simulink model "PubIfDecisionLM_MDL"  (R2020b)
settings: configuration reference "DspaceConfig" (kept outside this file)
PostLoadFcn:
  | if any(exist('dsrtsu_mdlpostloadfcn', 'file') ~= 0), dsrtsu_mdlpostloadfcn('Execute', bdroot); end
InitFcn:
  | , if any(exist('dsmpb_private', 'file') ~= 0), dsmpb_private('dsmpb_mdlclblib', 'Init', bdroot); end,
undefined symbols (not defined in the file or in its folder): OFM_OBJ_FUSIONTYPE_E, OFM_OBJ_MOVINGSTATE_E, OFM_OBJ_ORIENTATION_E, OFM_OBJ_TYPE_E, P_LM_Cyc, P_LM_EMLHistKapRcdBufSize, P_LM_EMLHistTrajBaseDis, P_LM_EMLHistTrajPNum, P_LM_EMLKapCorrMaxThre, P_LM_EMLMinKapThre, P_LM_EMLPathDisDiffThre, P_LM_EMLQuaFiltPar, P_LM_EMLTurnActKapThre, P_LM_EMLValidQuaThre, P_LM_FntPath1Disgap, P_LM_FntPath1MinDis, P_LM_FntPath1Timegap, P_LM_FntPath2Disgap, P_LM_FntPath2MinDis, P_LM_FntPath2Timegap, P_LM_FntPath3Disgap, P_LM_FntPath3MinDis, P_LM_FntPath3Timegap, P_LM_FusBLParFiltP, P_LM_FusEVDifC2Thre, P_LM_FusEVOPath1AllVSLDisThre, P_LM_FusEVOPath1AllVSLLostNumThre, P_LM_FusEVOPath1AllVSLQuaThre, P_LM_FusEVOPath1OTLFacNLC, P_LM_FusOTLQuaThre, P_LM_FusOTLSW, P_LM_FusParC0Index, P_LM_FusParC1Index, P_LM_FusParC2Index, P_LM_FusParC3Index, P_LM_FusVSLQuaThre, P_LM_FusVSLSW, P_LM_FusVSLValidSteerWheerAngThre, P_LM_FusVSLValidVxvThre, P_LM_LaneWidth, P_LM_OTLBufTPInfoEvaFactor, P_LM_OTLObjNum, P_LM_OTLObjSelectAgeThre, P_LM_OTLObjSelectDxAssessVx, P_LM_OTLObjSelectDxThre, P_LM_OTLObjSelectVxThre, P_LM_OTLObjSelectVyAssessDx, P_LM_OTLObjSelectVyThre, P_LM_OTLTrajPntBaseDis, P_LM_OTLTrajStdThre, P_LM_VSLAvailLineNum, P_LM_VSLBLSDiffThre, P_LM_VSLBLSDisRatio, P_LM_VSLFusBLParFiltP_C1, P_LM_VSLFusBLParFiltP_C2, P_LM_VSLFusBLParFiltP_C3, P_LM_VSLFusBLParFiltP_Quality, P_LM_VSLHistTrajBaseDis, P_LM_VSLHistTrajPNum, P_LM_VSLLCC0diff ... (+18)
libraries: simulink x145, LM_LIB x43
(part 8 of 24)

== system PubIfDecisionLM_MDL/Subsystem2/LM_Fusion1/LM_FusRatioCalc/LM_Fusion_EMLOnly/LM_FusEMLAndVSLRatioCalc ==
  Bus Creator : BusCreator  Inputs=15  OutDataTypeStr=Bus: LM_FusFntPathKInfoBus  NonVirtualBus=on
  Bus Creator1 : BusCreator  Inputs=6  OutDataTypeStr=Bus: LM_FusRearPathKInfoBus  NonVirtualBus=on
  Constant : Constant  OutDataTypeStr=single
  Constant1 : Constant  OutDataTypeStr=single
  Constant{3..14} (12 alike) : Constant  Value=0  OutDataTypeStr=single
  Constant2 : Constant  OutDataTypeStr=single
  LM_Fusion_RearPathK : Subsystem
  LM_FusFntPathK : Outport
  LM_FusRearPathK : Outport  Port=2
  wires:
  Constant9/1 -> Bus Creator/9  "LM_FusFntPath2RELK"
  Constant1/1 -> Bus Creator/6  "LM_FusFntPath2EMLK"
  Constant6/1 -> Bus Creator/5  "LM_FusFntPath1MALK"
  Constant10/1 -> Bus Creator/10  "LM_FusFntPath2MALK"
  Constant7/1 -> Bus Creator/7  "LM_FusFntPath2VSLK"
  Constant8/1 -> Bus Creator/8  "LM_FusFntPath2OTLK"
  Constant/1 -> Bus Creator/1  "LM_FusFntPath1EMLK"
  Constant3/1 -> Bus Creator/2  "LM_FusFntPath1VSLK"
  Constant14/1 -> Bus Creator/14  "LM_FusFntPath3RELK"
  Constant12/1 -> Bus Creator/12  "LM_FusFntPath3VSLK"
  Constant4/1 -> Bus Creator/3  "LM_FusFntPath1OTLK"
  Constant11/1 -> Bus Creator/15  "LM_FusFntPath3MALK"
  Constant5/1 -> Bus Creator/4  "LM_FusFntPath1RELK"
  Constant13/1 -> Bus Creator/13  "LM_FusFntPath3OTLK"
  Constant2/1 -> Bus Creator/11  "LM_FusFntPath3EMLK"
  Bus Creator1/1 -> LM_FusRearPathK/1  "LM_FusRearPathK"
  LM_Fusion_RearPathK/1(LM_FusRearPath1VSLK) -> Bus Creator1/1
  LM_Fusion_RearPathK/4(LM_FusRearPath1EMLK) -> Bus Creator1/4
  LM_Fusion_RearPathK/3(LM_FusRearPath3VSLK) -> Bus Creator1/3
  LM_Fusion_RearPathK/2(LM_FusRearPath2VSLK) -> Bus Creator1/2
  LM_Fusion_RearPathK/5(LM_FusRearPath2EMLK) -> Bus Creator1/5
  LM_Fusion_RearPathK/6(LM_FusRearPath3EMLK) -> Bus Creator1/6
  Bus Creator/1 -> LM_FusFntPathK/1  "LM_FusFntPathK"

== system PubIfDecisionLM_MDL/Subsystem2/LM_Fusion1/LM_FusRatioCalc/LM_Fusion_EO/LM_FusBaseLineC0Info ==
  LM_VSLLLC0Adju : Inport
  LM_VSLLRC0Adju : Inport  Port=2
  LM_VSLRLC0Adju : Inport  Port=3
  LM_VSLRRC0Adju : Inport  Port=4
  Signal Conversion{,1..3} (4 alike) : SignalConversion  OverrideOpt=off
  LM_LLC0 : Outport
  LM_LRC0 : Outport  Port=2
  LM_RLC0 : Outport  Port=3
  LM_RRC0 : Outport  Port=4
  wires:
  Signal Conversion3/1 -> LM_RRC0/1  "LM_RRC0"
  Signal Conversion2/1 -> LM_RLC0/1  "LM_RLC0"
  Signal Conversion1/1 -> LM_LRC0/1  "LM_LRC0"
  Signal Conversion/1 -> LM_LLC0/1  "LM_LLC0"
  LM_VSLRRC0Adju/1 -> Signal Conversion3/1
  LM_VSLRLC0Adju/1 -> Signal Conversion2/1
  LM_VSLLRC0Adju/1 -> Signal Conversion1/1
  LM_VSLLLC0Adju/1 -> Signal Conversion/1

== system PubIfDecisionLM_MDL/Subsystem2/LM_Fusion1/LM_FusRatioCalc/LM_Fusion_EO/LM_FusEVORatioCalc ==
  DIR_BUS : Inport
  LM_EML : Inport  Port=2
  LM_OTL : Inport  Port=3
  LM_Com : Inport  Port=4
  LM_VIE_BUS : Inport  Port=5
  Bus Creator : BusCreator  Inputs=15  OutDataTypeStr=Bus: LM_FusFntPathKInfoBus  NonVirtualBus=on
  Bus Creator1 : BusCreator  Inputs=6  OutDataTypeStr=Bus: LM_FusRearPathKInfoBus  NonVirtualBus=on
  Bus Selector : BusSelector  OutputSignals=LM_EMLFntPath1Quality,LM_EMLFntPath2Quality,LM_EMLFntPath3Quality
  Bus Selector1 : BusSelector  OutputSignals=LM_DIRTurnLeftValid,LM_DIRTurnRightValid,DIR_LC2LeValid,DIR_LC2RigValid
  Bus Selector3 : BusSelector  OutputSignals=LM_OTLFntPath1Qulity,LM_OTLFntPath2Qulity,LM_OTLFntPath3Qulity
  Bus Selector4 : BusSelector  OutputSignals=vxvRefMs
  LM_Fusion_FntPathK : Subsystem
  LM_Fusion_RearPathK : Subsystem
  Signal Conversion{,1..14} (15 alike) : SignalConversion  OverrideOpt=off
  LM_FusFntPathK : Outport
  LM_FusRearPathK : Outport  Port=2
  wires:
  Bus Selector4/1 -> LM_Fusion_FntPathK/7(vxvRefMs)  "<vxvRefMs>"
  LM_VIE_BUS/1 -> Bus Selector4/1
  Bus Selector3/3 -> LM_Fusion_FntPathK/6(LM_OTLFntPath3Qulity)  "<LM_OTLFntPath3Qulity>"
  Bus Selector3/2 -> LM_Fusion_FntPathK/5(LM_OTLFntPath2Qulity)  "<LM_OTLFntPath2Qulity>"
  Bus Selector3/1 -> LM_Fusion_FntPathK/4(LM_OTLFntPath1Qulity)  "<LM_OTLFntPath1Qulity>"
  Bus Selector/3 -> LM_Fusion_FntPathK/3(LM_EMLFntPath3Quality)  "<LM_EMLFntPath3Quality>"
  Bus Selector/2 -> LM_Fusion_FntPathK/2(LM_EMLFntPath2Quality)  "<LM_EMLFntPath2Quality>"
  Bus Selector/1 -> LM_Fusion_FntPathK/1(LM_EMLFntPath1Quality)  "<LM_EMLFntPath1Quality>"
  LM_OTL/1 -> Bus Selector3/1
  LM_EML/1 -> Bus Selector/1
  Bus Creator1/1 -> LM_FusRearPathK/1  "LM_FusRearPathK"
  LM_Fusion_RearPathK/1(LM_FusRearPath1VSLK) -> Bus Creator1/1
  LM_Fusion_RearPathK/4(LM_FusRearPath1EMLK) -> Bus Creator1/4
  LM_Fusion_RearPathK/3(LM_FusRearPath3VSLK) -> Bus Creator1/3
  LM_Fusion_RearPathK/2(LM_FusRearPath2VSLK) -> Bus Creator1/2
  LM_Fusion_RearPathK/5(LM_FusRearPath2EMLK) -> Bus Creator1/5
  LM_Fusion_RearPathK/6(LM_FusRearPath3EMLK) -> Bus Creator1/6
  Bus Creator/1 -> LM_FusFntPathK/1  "LM_FusFntPathK"
  LM_Fusion_FntPathK/1(LM_FusEOFntPath1EMLK) -> Signal Conversion/1
  LM_Fusion_FntPathK/2(LM_FusEOFntPath1VSLK) -> Signal Conversion1/1
  LM_Fusion_FntPathK/3(LM_FusEOFntPath1OTLK) -> Signal Conversion2/1
  LM_Fusion_FntPathK/4(LM_FusEOFntPath1RELK) -> Signal Conversion3/1
  LM_Fusion_FntPathK/5(LM_FusEOFntPath1MALK) -> Signal Conversion4/1
  LM_Fusion_FntPathK/6(LM_FusEOFntPath2EMLK) -> Signal Conversion5/1
  LM_Fusion_FntPathK/7(LM_FusEOFntPath2VSLK) -> Signal Conversion6/1
  LM_Fusion_FntPathK/8(LM_FusEOFntPath2OTLK) -> Signal Conversion7/1
  LM_Fusion_FntPathK/9(LM_FusEOFntPath2RELK) -> Signal Conversion8/1
  LM_Fusion_FntPathK/10(LM_FusEOFntPath2MALK) -> Signal Conversion9/1
  LM_Fusion_FntPathK/11(LM_FusEOFntPath3EMLK) -> Signal Conversion10/1
  LM_Fusion_FntPathK/12(LM_FusEOFntPath3VSLK) -> Signal Conversion11/1
  LM_Fusion_FntPathK/13(LM_FusEOFntPath3OTLK) -> Signal Conversion12/1
  LM_Fusion_FntPathK/14(LM_FusEOFntPath3RELK) -> Signal Conversion13/1
  LM_Fusion_FntPathK/15(LM_FusEOFntPath3MALK) -> Signal Conversion14/1
  Signal Conversion/1 -> Bus Creator/1  "LM_FusFntPath1EMLK"
  Signal Conversion1/1 -> Bus Creator/2  "LM_FusFntPath1VSLK"
  Signal Conversion2/1 -> Bus Creator/3  "LM_FusFntPath1OTLK"
  Signal Conversion3/1 -> Bus Creator/4  "LM_FusFntPath1RELK"
  Signal Conversion4/1 -> Bus Creator/5  "LM_FusFntPath1MALK"
  Signal Conversion7/1 -> Bus Creator/8  "LM_FusFntPath2OTLK"
  Signal Conversion6/1 -> Bus Creator/7  "LM_FusFntPath2VSLK"
  Signal Conversion8/1 -> Bus Creator/9  "LM_FusFntPath2RELK"
  Signal Conversion9/1 -> Bus Creator/10  "LM_FusFntPath2MALK"
  Signal Conversion5/1 -> Bus Creator/6  "LM_FusFntPath2EMLK"
  Signal Conversion11/1 -> Bus Creator/12  "LM_FusFntPath3VSLK"
  Signal Conversion10/1 -> Bus Creator/11  "LM_FusFntPath3EMLK"
  Signal Conversion12/1 -> Bus Creator/13  "LM_FusFntPath3OTLK"
  Signal Conversion13/1 -> Bus Creator/14  "LM_FusFntPath3RELK"
  Signal Conversion14/1 -> Bus Creator/15  "LM_FusFntPath3MALK"
  DIR_BUS/1 -> Bus Selector1/1
  Bus Selector1/2 -> LM_Fusion_FntPathK/9(DIR_TurnRightValid)  "<LM_DIRTurnRightValid>"
  Bus Selector1/1 -> LM_Fusion_FntPathK/8(DIR_TurnLeftValid)  "<LM_DIRTurnLeftValid>"
  Bus Selector1/3 -> LM_Fusion_FntPathK/10(DIR_LC2LeValid)  "<DIR_LC2LeValid>"
  Bus Selector1/4 -> LM_Fusion_FntPathK/11(DIR_LC2RigValid)  "<DIR_LC2RigValid>"

== system PubIfDecisionLM_MDL/Subsystem2/LM_Fusion1/LM_FusRatioCalc/LM_Fusion_EV/LM_FusBaseLineC0Info ==
  LM_FusFntPathK : Inport
  LM_VSL : Inport  Port=2
  LM_EML : Inport  Port=3
  Bus Selector : BusSelector  OutputSignals=LM_VSLLLC0,LM_VSLLRC0,LM_VSLRLC0,LM_VSLRRC0
  Bus Selector1 : BusSelector  OutputSignals=LM_FusFntPath1EMLK
  Bus Selector2 : BusSelector  OutputSignals=LM_EMLLLC0,LM_EMLLRC0,LM_EMLRLC0,LM_EMLRRC0
  Constant : Constant  OutDataTypeStr=single
  If : If  IfExpression=u1 ~= 0
  If Action Subsystem : Subsystem  TreatAsAtomicUnit=on
  If Action Subsystem1 : Subsystem  TreatAsAtomicUnit=on
  Merge{,1..3} (4 alike) : Merge
  Relational Operator : RelationalOperator  Operator===  OutDataTypeStr=boolean  RndMeth=Simplest
  LM_LLC0 : Outport
  LM_LRC0 : Outport  Port=2
  LM_RLC0 : Outport  Port=3
  LM_RRC0 : Outport  Port=4
  wires:
  LM_FusFntPathK/1 -> Bus Selector1/1
  Bus Selector1/1 -> Relational Operator/1  "<LM_FusFntPath1EMLK>"
  Relational Operator/1 -> If/1
  If/1 -> If Action Subsystem/Action
  If/2 -> If Action Subsystem1/Action
  Bus Selector/1 -> If Action Subsystem1/1(LM_VSLLLC0Adju)  "<LM_VSLLLC0>"
  Bus Selector/2 -> If Action Subsystem1/2(LM_VSLLRC0Adju)  "<LM_VSLLRC0>"
  Bus Selector/3 -> If Action Subsystem1/3(LM_VSLRLC0Adju)  "<LM_VSLRLC0>"
  Bus Selector/4 -> If Action Subsystem1/4(LM_VSLRRC0Adju)  "<LM_VSLRRC0>"
  LM_VSL/1 -> Bus Selector/1
  Bus Selector2/1 -> If Action Subsystem/1(LM_EMLLLC0Adju)  "<LM_EMLLLC0>"
  Bus Selector2/2 -> If Action Subsystem/2(LM_EMLLRC0Adju)  "<LM_EMLLRC0>"
  Bus Selector2/3 -> If Action Subsystem/3(LM_EMLRLC0Adju)  "<LM_EMLRLC0>"
  Bus Selector2/4 -> If Action Subsystem/4(LM_EMLRRC0Adju)  "<LM_EMLRRC0>"
  LM_EML/1 -> Bus Selector2/1
  If Action Subsystem/1(LM_LLC0) -> Merge/1
  If Action Subsystem1/1(LM_LLC0) -> Merge/2
  If Action Subsystem/2(LM_LRC0) -> Merge1/1
  If Action Subsystem1/2(LM_LRC0) -> Merge1/2
  If Action Subsystem/3(LM_RLC0) -> Merge2/1
  If Action Subsystem1/3(LM_RLC0) -> Merge2/2
  If Action Subsystem/4(LM_RRC0) -> Merge3/1
  If Action Subsystem1/4(LM_RRC0) -> Merge3/2
  Merge/1 -> LM_LLC0/1  "LM_LLC0"
  Merge1/1 -> LM_LRC0/1  "LM_LRC0"
  Merge2/1 -> LM_RLC0/1  "LM_RLC0"
  Merge3/1 -> LM_RRC0/1  "LM_RRC0"
  Constant/1 -> Relational Operator/2

== system PubIfDecisionLM_MDL/Subsystem2/LM_Fusion1/LM_FusRatioCalc/LM_Fusion_EV/LM_FusEMLAndVSLRatioCalc ==
  LM_VIE_BUS : Inport
  LM_ComBus : Inport  Port=2
  DIR_BUS : Inport  Port=3
  LM_VSL : Inport  Port=4
  LM_EML : Inport  Port=5
  Bus Creator : BusCreator  Inputs=15  OutDataTypeStr=Bus: LM_FusFntPathKInfoBus  NonVirtualBus=on
  Bus Creator1 : BusCreator  Inputs=6  OutDataTypeStr=Bus: LM_FusRearPathKInfoBus  NonVirtualBus=on
  Bus Selector : BusSelector  OutputSignals=LM_VSLFntPath1Quality,LM_VSLFntPath2Quality,LM_VSLFntPath3Quality,LM_VSLFntPath1P,LM_VSLBaseDis
  Bus Selector1 : BusSelector  OutputSignals=LM_EMLFntPath1Quality,LM_EMLFntPath2Quality,LM_EMLFntPath3Quality,LM_EMLFntPath1P
  Bus Selector2 : BusSelector  OutputSignals=LM_ComLineLostNum
  Bus Selector3 : BusSelector  OutputSignals=LM_DIRTurnLeftValid,LM_DIRTurnRightValid,DIR_LC2LeValid,DIR_LC2RigValid
  Bus Selector4 : BusSelector  OutputSignals=vxvRefMs
  LM_Fusion_FntPathK : Subsystem
  LM_Fusion_RearPathK : Subsystem
  Signal Conversion{,1..14} (15 alike) : SignalConversion  OverrideOpt=off
  LM_FusFntPathK : Outport
  LM_FusRearPathK : Outport  Port=2
  wires:
  Bus Selector/5 -> LM_Fusion_FntPathK/5(LM_VSLBaseDis)  "<LM_VSLBaseDis>"
  Bus Selector/3 -> LM_Fusion_FntPathK/3(LM_VSLFntPath3Quality)  "<LM_VSLFntPath3Quality>"
  Bus Selector1/2 -> LM_Fusion_FntPathK/7(LM_EMLFntPath2Quality)  "<LM_EMLFntPath2Quality>"
  Bus Selector1/1 -> LM_Fusion_FntPathK/6(LM_EMLFntPath1Quality)  "<LM_EMLFntPath1Quality>"
  LM_VSL/1 -> Bus Selector/1
  LM_EML/1 -> Bus Selector1/1
  Bus Selector/1 -> LM_Fusion_FntPathK/1(LM_VSLFntPath1Quality)  "<LM_VSLFntPath1Quality>"
  Bus Selector/4 -> LM_Fusion_FntPathK/4(LM_VSLFntPath1P)  "<LM_VSLFntPath1P>"
  Bus Selector/2 -> LM_Fusion_FntPathK/2(LM_VSLFntPath2Quality)  "<LM_VSLFntPath2Quality>"
  Bus Selector1/3 -> LM_Fusion_FntPathK/8(LM_EMLFntPath3Quality)  "<LM_EMLFntPath3Quality>"
  LM_ComBus/1 -> Bus Selector2/1
  Bus Selector1/4 -> LM_Fusion_FntPathK/9(LM_EMLFntPath1P)  "<LM_EMLFntPath1P>"
  Bus Creator/1 -> LM_FusFntPathK/1  "LM_FusFntPathK"
  LM_Fusion_RearPathK/6(LM_FusRearPath3EMLK) -> Bus Creator1/6
  LM_Fusion_RearPathK/5(LM_FusRearPath2EMLK) -> Bus Creator1/5
  LM_Fusion_RearPathK/2(LM_FusRearPath2VSLK) -> Bus Creator1/2
  LM_Fusion_RearPathK/3(LM_FusRearPath3VSLK) -> Bus Creator1/3
  LM_Fusion_RearPathK/4(LM_FusRearPath1EMLK) -> Bus Creator1/4
  LM_Fusion_RearPathK/1(LM_FusRearPath1VSLK) -> Bus Creator1/1
  Bus Creator1/1 -> LM_FusRearPathK/1  "LM_FusRearPathK"
  Bus Selector2/1 -> LM_Fusion_FntPathK/10(LM_ComLineLostNum)  "<LM_ComLineLostNum>"
  LM_Fusion_FntPathK/1(LM_FusEVFntPath1EMLK) -> Signal Conversion/1
  LM_Fusion_FntPathK/2(LM_FusEVFntPath1VSLK) -> Signal Conversion1/1
  LM_Fusion_FntPathK/3(LM_FusEVFntPath1OTLK) -> Signal Conversion2/1
  LM_Fusion_FntPathK/4(LM_FusEVFntPath1RELK) -> Signal Conversion3/1
  LM_Fusion_FntPathK/5(LM_FusEVFntPath1MALK) -> Signal Conversion4/1
  LM_Fusion_FntPathK/6(LM_FusEVFntPath2EMLK) -> Signal Conversion5/1
  LM_Fusion_FntPathK/7(LM_FusEVFntPath2VSLK) -> Signal Conversion6/1
  LM_Fusion_FntPathK/8(LM_FusEVFntPath2OTLK) -> Signal Conversion7/1
  LM_Fusion_FntPathK/9(LM_FusEVFntPath2RELK) -> Signal Conversion8/1
  LM_Fusion_FntPathK/10(LM_FusEVFntPath2MALK) -> Signal Conversion9/1
  LM_Fusion_FntPathK/11(LM_FusEVFntPath3EMLK) -> Signal Conversion10/1
  LM_Fusion_FntPathK/12(LM_FusEVFntPath3VSLK) -> Signal Conversion11/1
  LM_Fusion_FntPathK/13(LM_FusEVFntPath3OTLK) -> Signal Conversion12/1
  LM_Fusion_FntPathK/14(LM_FusEVFntPath3RELK) -> Signal Conversion13/1
  LM_Fusion_FntPathK/15(LM_FusEVFntPath3MALK) -> Signal Conversion14/1
  Signal Conversion10/1 -> Bus Creator/11  "LM_FusFntPath3EMLK"
  Signal Conversion12/1 -> Bus Creator/13  "LM_FusFntPath3OTLK"
  Signal Conversion3/1 -> Bus Creator/4  "LM_FusFntPath1RELK"
  Signal Conversion14/1 -> Bus Creator/15  "LM_FusFntPath3MALK"
  Signal Conversion2/1 -> Bus Creator/3  "LM_FusFntPath1OTLK"
  Signal Conversion11/1 -> Bus Creator/12  "LM_FusFntPath3VSLK"
  Signal Conversion13/1 -> Bus Creator/14  "LM_FusFntPath3RELK"
  Signal Conversion1/1 -> Bus Creator/2  "LM_FusFntPath1VSLK"
  Signal Conversion/1 -> Bus Creator/1  "LM_FusFntPath1EMLK"
  Signal Conversion7/1 -> Bus Creator/8  "LM_FusFntPath2OTLK"
  Signal Conversion6/1 -> Bus Creator/7  "LM_FusFntPath2VSLK"
  Signal Conversion9/1 -> Bus Creator/10  "LM_FusFntPath2MALK"
  Signal Conversion4/1 -> Bus Creator/5  "LM_FusFntPath1MALK"
  Signal Conversion5/1 -> Bus Creator/6  "LM_FusFntPath2EMLK"
  Signal Conversion8/1 -> Bus Creator/9  "LM_FusFntPath2RELK"
  DIR_BUS/1 -> Bus Selector3/1
  Bus Selector3/1 -> LM_Fusion_FntPathK/11(DIR_TurnLeftValid)  "<LM_DIRTurnLeftValid>"
  Bus Selector3/2 -> LM_Fusion_FntPathK/12(DIR_TurnRightValid)  "<LM_DIRTurnRightValid>"
  Bus Selector3/3 -> LM_Fusion_FntPathK/13(DIR_LC2LeValid)  "<DIR_LC2LeValid>"
  Bus Selector3/4 -> LM_Fusion_FntPathK/14(DIR_LC2RigValid)  "<DIR_LC2RigValid>"
  LM_VIE_BUS/1 -> Bus Selector4/1
  Bus Selector4/1 -> LM_Fusion_FntPathK/15(vxvRefMs)  "<vxvRefMs>"

== system PubIfDecisionLM_MDL/Subsystem2/LM_Fusion1/LM_FusRatioCalc/LM_Fusion_EVO/LM_FusBaseLineC0Info ==
  LM_VSLLLC0Adju : Inport
  LM_VSLLRC0Adju : Inport  Port=2
  LM_VSLRLC0Adju : Inport  Port=3
  LM_VSLRRC0Adju : Inport  Port=4
  Signal Conversion{,1..3} (4 alike) : SignalConversion  OverrideOpt=off
  LM_LLC0 : Outport
  LM_LRC0 : Outport  Port=2
  LM_RLC0 : Outport  Port=3
  LM_RRC0 : Outport  Port=4
  wires:
  LM_VSLLLC0Adju/1 -> Signal Conversion/1
  LM_VSLLRC0Adju/1 -> Signal Conversion1/1
  LM_VSLRLC0Adju/1 -> Signal Conversion2/1
  LM_VSLRRC0Adju/1 -> Signal Conversion3/1
  Signal Conversion/1 -> LM_LLC0/1  "LM_LLC0"
  Signal Conversion1/1 -> LM_LRC0/1  "LM_LRC0"
  Signal Conversion2/1 -> LM_RLC0/1  "LM_RLC0"
  Signal Conversion3/1 -> LM_RRC0/1  "LM_RRC0"

== system PubIfDecisionLM_MDL/Subsystem2/LM_Fusion1/LM_FusRatioCalc/LM_Fusion_EVO/LM_FusEVORatioCalc ==
  LM_VSL : Inport
  LM_EML : Inport  Port=2
  LM_OTL : Inport  Port=3
  LM_Com : Inport  Port=4
  LM_VIE_BUS : Inport  Port=5
  DIR_BUS : Inport  Port=6
  Bus Creator : BusCreator  Inputs=15  OutDataTypeStr=Bus: LM_FusFntPathKInfoBus  NonVirtualBus=on
  Bus Creator1 : BusCreator  Inputs=6  OutDataTypeStr=Bus: LM_FusRearPathKInfoBus  NonVirtualBus=on
  Bus Selector : BusSelector  OutputSignals=LM_EMLFntPath1Quality,LM_EMLFntPath2Quality,LM_EMLFntPath3Quality
  Bus Selector1 : BusSelector  OutputSignals=LM_VSLFntPath1Quality,LM_VSLFntPath2Quality,LM_VSLFntPath3Quality,LM_VSLBaseDis
  Bus Selector2 : BusSelector  OutputSignals=LM_ComLineLostNum,LM_PathDisBus.LM_FntPath1Dis,LM_PathDisBus.LM_FntPath2Dis
  Bus Selector3 : BusSelector  OutputSignals=LM_OTLFntPath1Qulity,LM_OTLFntPath2Qulity,LM_OTLFntPath3Qulity
  Bus Selector4 : BusSelector  OutputSignals=vxvRefMs
  Bus Selector5 : BusSelector  OutputSignals=LM_DIRTurnLeftValid,LM_DIRTurnRightValid,DIR_LC2LeValid,DIR_LC2RigValid
  LM_Fusion_FntPathK : Subsystem
  LM_Fusion_RearPathK : Subsystem
  Signal Conversion{,1..14} (15 alike) : SignalConversion  OverrideOpt=off
  LM_FusFntPathK : Outport
  LM_FusRearPathK : Outport  Port=2
  wires:
  Bus Creator/1 -> LM_FusFntPathK/1  "LM_FusFntPathK"
  LM_Fusion_RearPathK/6(LM_FusRearPath3EMLK) -> Bus Creator1/6
  LM_Fusion_RearPathK/5(LM_FusRearPath2EMLK) -> Bus Creator1/5
  LM_Fusion_RearPathK/2(LM_FusRearPath2VSLK) -> Bus Creator1/2
  LM_Fusion_RearPathK/3(LM_FusRearPath3VSLK) -> Bus Creator1/3
  LM_Fusion_RearPathK/4(LM_FusRearPath1EMLK) -> Bus Creator1/4
  LM_Fusion_RearPathK/1(LM_FusRearPath1VSLK) -> Bus Creator1/1
  Bus Creator1/1 -> LM_FusRearPathK/1  "LM_FusRearPathK"
  LM_VSL/1 -> Bus Selector1/1
  LM_EML/1 -> Bus Selector/1
  LM_OTL/1 -> Bus Selector3/1
  LM_Com/1 -> Bus Selector2/1
  Bus Selector/1 -> LM_Fusion_FntPathK/1(LM_EMLFntPath1Quality)  "<LM_EMLFntPath1Quality>"
  Bus Selector/2 -> LM_Fusion_FntPathK/2(LM_EMLFntPath2Quality)  "<LM_EMLFntPath2Quality>"
  Bus Selector/3 -> LM_Fusion_FntPathK/3(LM_EMLFntPath3Quality)  "<LM_EMLFntPath3Quality>"
  Bus Selector1/1 -> LM_Fusion_FntPathK/4(LM_VSLFntPath1Quality)  "<LM_VSLFntPath1Quality>"
  Bus Selector1/2 -> LM_Fusion_FntPathK/5(LM_VSLFntPath2Quality)  "<LM_VSLFntPath2Quality>"
  Bus Selector1/3 -> LM_Fusion_FntPathK/6(LM_VSLFntPath3Quality)  "<LM_VSLFntPath3Quality>"
  Bus Selector1/4 -> LM_Fusion_FntPathK/7(LM_VSLBaseDis)  "<LM_VSLBaseDis>"
  Bus Selector3/1 -> LM_Fusion_FntPathK/8(LM_OTLFntPath1Qulity)  "<LM_OTLFntPath1Qulity>"
  Bus Selector2/1 -> LM_Fusion_FntPathK/11(LM_ComLineLostNum)  "<LM_ComLineLostNum>"
  Bus Selector3/2 -> LM_Fusion_FntPathK/9(LM_OTLFntPath2Qulity)  "<LM_OTLFntPath2Qulity>"
  Bus Selector3/3 -> LM_Fusion_FntPathK/10(LM_OTLFntPath3Qulity)  "<LM_OTLFntPath3Qulity>"
  Bus Selector2/2 -> LM_Fusion_FntPathK/12(LM_FntPath1Dis)  "<LM_FntPath1Dis>"
  LM_VIE_BUS/1 -> Bus Selector4/1
  Bus Selector4/1 -> LM_Fusion_FntPathK/14(vxvRefMs)  "<vxvRefMs>"
  Signal Conversion8/1 -> Bus Creator/9  "LM_FusFntPath2RELK"
  Signal Conversion5/1 -> Bus Creator/6  "LM_FusFntPath2EMLK"
  Signal Conversion4/1 -> Bus Creator/5  "LM_FusFntPath1MALK"
  Signal Conversion9/1 -> Bus Creator/10  "LM_FusFntPath2MALK"
  Signal Conversion6/1 -> Bus Creator/7  "LM_FusFntPath2VSLK"
  Signal Conversion7/1 -> Bus Creator/8  "LM_FusFntPath2OTLK"
  Signal Conversion/1 -> Bus Creator/1  "LM_FusFntPath1EMLK"
  Signal Conversion1/1 -> Bus Creator/2  "LM_FusFntPath1VSLK"
  Signal Conversion13/1 -> Bus Creator/14  "LM_FusFntPath3RELK"
  Signal Conversion11/1 -> Bus Creator/12  "LM_FusFntPath3VSLK"
  Signal Conversion2/1 -> Bus Creator/3  "LM_FusFntPath1OTLK"
  Signal Conversion14/1 -> Bus Creator/15  "LM_FusFntPath3MALK"
  Signal Conversion3/1 -> Bus Creator/4  "LM_FusFntPath1RELK"
  Signal Conversion12/1 -> Bus Creator/13  "LM_FusFntPath3OTLK"
  Signal Conversion10/1 -> Bus Creator/11  "LM_FusFntPath3EMLK"
  LM_Fusion_FntPathK/15(LM_FusEVOFntPath3MALK) -> Signal Conversion14/1
  LM_Fusion_FntPathK/14(LM_FusEVOFntPath3RELK) -> Signal Conversion13/1
  LM_Fusion_FntPathK/13(LM_FusEVOFntPath3OTLK) -> Signal Conversion12/1
  LM_Fusion_FntPathK/12(LM_FusEVOFntPath3VSLK) -> Signal Conversion11/1
  LM_Fusion_FntPathK/11(LM_FusEVOFntPath3EMLK) -> Signal Conversion10/1
  LM_Fusion_FntPathK/10(LM_FusEVOFntPath2MALK) -> Signal Conversion9/1
  LM_Fusion_FntPathK/9(LM_FusEVOFntPath2RELK) -> Signal Conversion8/1
  LM_Fusion_FntPathK/8(LM_FusEVOFntPath2OTLK) -> Signal Conversion7/1
  LM_Fusion_FntPathK/7(LM_FusEVOFntPath2VSLK) -> Signal Conversion6/1
  LM_Fusion_FntPathK/6(LM_FusEVOFntPath2EMLK) -> Signal Conversion5/1
  LM_Fusion_FntPathK/5(LM_FusEVOFntPath1MALK) -> Signal Conversion4/1
  LM_Fusion_FntPathK/4(LM_FusEVOFntPath1RELK) -> Signal Conversion3/1
  LM_Fusion_FntPathK/3(LM_FusEVOFntPath1OTLK) -> Signal Conversion2/1
  LM_Fusion_FntPathK/2(LM_FusEVOFntPath1VSLK) -> Signal Conversion1/1
  LM_Fusion_FntPathK/1(LM_FusEVOFntPath1EMLK) -> Signal Conversion/1
  DIR_BUS/1 -> Bus Selector5/1
  Bus Selector5/1 -> LM_Fusion_FntPathK/15(DIR_TurnLeftValid)  "<LM_DIRTurnLeftValid>"
  Bus Selector5/2 -> LM_Fusion_FntPathK/16(DIR_TurnRightValid)  "<LM_DIRTurnRightValid>"
  Bus Selector5/3 -> LM_Fusion_FntPathK/17(DIR_LC2LeValid)  "<DIR_LC2LeValid>"
  Bus Selector5/4 -> LM_Fusion_FntPathK/18(DIR_LC2RigValid)  "<DIR_LC2RigValid>"
  Bus Selector2/3 -> LM_Fusion_FntPathK/13(LM_FntPath2Dis)  "<LM_FntPath2Dis>"

== system PubIfDecisionLM_MDL/Subsystem2/LM_Fusion1/LM_Fus_BLConnectivityCheck/LM_Fus_BLFntPahtConnectivityCheck/LM_Fus_BLFntPahtConnectivityCheck ==
  LM_FusBLFntPath1C0 : Inport
  LM_FusBLFntPath1C1 : Inport  Port=2
  LM_FusBLFntPath1C2 : Inport  Port=3
  LM_FusBLFntPath1C3 : Inport  Port=4
  LM_FusBLFntPath1Quality : Inport  Port=5
  LM_FusBLFntPath2C0BefAduj : Inport  Port=6
  LM_FusBLFntPath2C1 : Inport  Port=7
  LM_FusBLFntPath2C2 : Inport  Port=8
  LM_FusBLFntPath2C3 : Inport  Port=9
  LM_FusBLFntPath2Quality : Inport  Port=10
  LM_FusBLFntPath3C0BefAduj : Inport  Port=11
  LM_FusBLFntPath3C1 : Inport  Port=12
  LM_FusBLFntPath3C2 : Inport  Port=13
  LM_FusBLFntPath3C3 : Inport  Port=14
  LM_FusBLFntPath3Quality : Inport  Port=15
  LM_FntPath1Dis : Inport  Port=16
  LM_FntPath2Dis : Inport  Port=17
  LM_Fus_BLFntPath1Info : Subsystem
  LM_Fus_BLFntPath2Info : Subsystem
  LM_Fus_BLFntPath3Info : Subsystem
  LM_FusBLFntPath1C0Adju : Outport
  LM_FusBLFntPath1C1Adju : Outport  Port=2
  LM_FusBLFntPath1C2Adju : Outport  Port=3
  LM_FusBLFntPath1C3Adju : Outport  Port=4
  LM_FusBLFntPath1QualityAdju : Outport  Port=5
  LM_FusBLFntPath2C0Adju : Outport  Port=6
  LM_FusBLFntPath2C1Adju : Outport  Port=7
  LM_FusBLFntPath2C2Adju : Outport  Port=8
  LM_FusBLFntPath2C3Adju : Outport  Port=9
  LM_FusBLFntPath2QualityAdju : Outport  Port=10
  LM_FusBLFntPath3C0Adju : Outport  Port=11
  LM_FusBLFntPath3C1Adju : Outport  Port=12
  LM_FusBLFntPath3C2Adju : Outport  Port=13
  LM_FusBLFntPath3C3Adju : Outport  Port=14
  LM_FusBLFntPath3QualityAdju : Outport  Port=15
  wires:
  LM_FusBLFntPath1Quality/1 -> LM_Fus_BLFntPath1Info/1(LM_FusBLFntPath1Quality)
  LM_FusBLFntPath1C0/1 -> LM_Fus_BLFntPath1Info/2(LM_FusBLFntPath1C0), LM_Fus_BLFntPath2Info/1(LM_FusBLFntPath1C0)
  LM_FusBLFntPath1C1/1 -> LM_Fus_BLFntPath1Info/3(LM_FusBLFntPath1C1), LM_Fus_BLFntPath2Info/2(LM_FusBLFntPath1C1)
  LM_FusBLFntPath1C2/1 -> LM_Fus_BLFntPath1Info/4(LM_FusBLFntPath1C2), LM_Fus_BLFntPath2Info/3(LM_FusBLFntPath1C2)
  LM_FusBLFntPath1C3/1 -> LM_Fus_BLFntPath1Info/5(LM_FusBLFntPath1C3), LM_Fus_BLFntPath2Info/4(LM_FusBLFntPath1C3)
  LM_FusBLFntPath2C0BefAduj/1 -> LM_Fus_BLFntPath2Info/6(LM_FusBLFntPath2C0BefAduj)
  LM_FusBLFntPath2C1/1 -> LM_Fus_BLFntPath2Info/7(LM_FusBLFntPath2C1), LM_Fus_BLFntPath3Info/2(LM_FusBLFntPath2C1)
  LM_FusBLFntPath2C2/1 -> LM_Fus_BLFntPath2Info/8(LM_FusBLFntPath2C2), LM_Fus_BLFntPath3Info/3(LM_FusBLFntPath2C2)
  LM_FusBLFntPath2C3/1 -> LM_Fus_BLFntPath2Info/9(LM_FusBLFntPath2C3), LM_Fus_BLFntPath3Info/4(LM_FusBLFntPath2C3)
  LM_FusBLFntPath2Quality/1 -> LM_Fus_BLFntPath2Info/5(LM_FusBLFntPath2Quality)
  LM_FntPath1Dis/1 -> LM_Fus_BLFntPath2Info/10(LM_FntPath1Dis)
  LM_FusBLFntPath3C0BefAduj/1 -> LM_Fus_BLFntPath3Info/5(LM_FusBLFntPath3C0BefAduj)
  LM_FusBLFntPath3C1/1 -> LM_Fus_BLFntPath3Info/6(LM_FusBLFntPath3C1)
  LM_FusBLFntPath3C2/1 -> LM_Fus_BLFntPath3Info/7(LM_FusBLFntPath3C2)
  LM_FusBLFntPath3C3/1 -> LM_Fus_BLFntPath3Info/8(LM_FusBLFntPath3C3)
  LM_FusBLFntPath3Quality/1 -> LM_Fus_BLFntPath3Info/9(LM_FusBLFntPath3Quality)
  LM_FntPath2Dis/1 -> LM_Fus_BLFntPath3Info/10(LM_FntPath2Dis)
  LM_Fus_BLFntPath1Info/1(LM_FusBLFntPath1C0Adju) -> LM_FusBLFntPath1C0Adju/1
  LM_Fus_BLFntPath1Info/2(LM_FusBLFntPath1C1Adju) -> LM_FusBLFntPath1C1Adju/1
  LM_Fus_BLFntPath1Info/3(LM_FusBLFntPath1C2Adju) -> LM_FusBLFntPath1C2Adju/1
  LM_Fus_BLFntPath1Info/4(LM_FusBLFntPath1C3Adju) -> LM_FusBLFntPath1C3Adju/1
  LM_Fus_BLFntPath1Info/5(LM_FusBLFntPath1QualityAdju) -> LM_FusBLFntPath1QualityAdju/1
  LM_Fus_BLFntPath2Info/5(LM_FusBLFntPath2QualityAdju) -> LM_FusBLFntPath2QualityAdju/1
  LM_Fus_BLFntPath2Info/4(LM_FusBLFntPath2C3Adju) -> LM_FusBLFntPath2C3Adju/1
  LM_Fus_BLFntPath2Info/3(LM_FusBLFntPath2C2Adju) -> LM_FusBLFntPath2C2Adju/1
  LM_Fus_BLFntPath2Info/2(LM_FusBLFntPath2C1Adju) -> LM_FusBLFntPath2C1Adju/1
  LM_Fus_BLFntPath2Info/1(LM_FusBLFntPath2C0Adju) -> LM_FusBLFntPath2C0Adju/1, [LM_FusBLFntPath2C0Adju]
  LM_Fus_BLFntPath3Info/1(LM_FusBLFntPath3C0Adju) -> LM_FusBLFntPath3C0Adju/1
  LM_Fus_BLFntPath3Info/2(LM_FusBLFntPath3C1Adju) -> LM_FusBLFntPath3C1Adju/1
  LM_Fus_BLFntPath3Info/3(LM_FusBLFntPath3C2Adju) -> LM_FusBLFntPath3C2Adju/1
  LM_Fus_BLFntPath3Info/4(LM_FusBLFntPath3C3Adju) -> LM_FusBLFntPath3C3Adju/1
  LM_Fus_BLFntPath3Info/5(LM_FusBLFntPath3QualityAdju) -> LM_FusBLFntPath3QualityAdju/1
  [LM_FusBLFntPath2C0Adju] -> LM_Fus_BLFntPath3Info/1(LM_FusBLFntPath2C0Aduj)

== system PubIfDecisionLM_MDL/Subsystem2/LM_Fusion1/LM_Fus_BLConnectivityCheck/LM_Fus_BLRearPahtConnectivityCheck/LM_Fus_BLRearPahtConnectivityCheck ==
  LM_FusBLRearPath1C0 : Inport
  LM_FusBLRearPath1C1 : Inport  Port=2
  LM_FusBLRearPath1C2 : Inport  Port=3
  LM_FusBLRearPath1C3 : Inport  Port=4
  LM_FusBLRearPath1Quality : Inport  Port=5
  LM_FusBLRearPath2C0BefAduj : Inport  Port=6
  LM_FusBLRearPath2C1 : Inport  Port=7
  LM_FusBLRearPath2C2 : Inport  Port=8
  LM_FusBLRearPath2C3 : Inport  Port=9
  LM_FusBLRearPath2Quality : Inport  Port=10
  LM_FusBLRearPath3C0BefAduj : Inport  Port=11
  LM_FusBRearPath3C1 : Inport  Port=12
  LM_FusBLRearPath3C2 : Inport  Port=13
  LM_FusBLRearPath3C3 : Inport  Port=14
  LM_FusBLRearPath3Quality : Inport  Port=15
  LM_RearPath1Dis : Inport  Port=16
  LM_RearPath2Dis : Inport  Port=17
  LM_Fus_BLFntPath2Info : Subsystem
  LM_Fus_BLFntPath3Info : Subsystem
  LM_Fus_BLRearPath1Info : Subsystem
  LM_FusBLRearPath1C0Adju : Outport
  LM_FusBLRearPath1C1Adju : Outport  Port=2
  LM_FusBLRearPath1C2Adju : Outport  Port=3
  LM_FusBLRearPath1C3Adju : Outport  Port=4
  LM_FusBLRearPath1QualityAdju : Outport  Port=5
  LM_FusBLRearPath2C0Adju : Outport  Port=6
  LM_FusBLRearPath2C1Adju : Outport  Port=7
  LM_FusBLRearPath2C2Adju : Outport  Port=8
  LM_FusBLRearPath2C3Adju : Outport  Port=9
  LM_FusBLRearPath2QualityAdju : Outport  Port=10
  LM_FusBLRearPath3C0Adju : Outport  Port=11
  LM_FusBLRearPath3C1Adju : Outport  Port=12
  LM_FusBLRearPath3C2Adju : Outport  Port=13
  LM_FusBLRearPath3C3Adju : Outport  Port=14
  LM_FusBLRearPath3QualityAdju : Outport  Port=15
  wires:
  LM_FusBLRearPath1Quality/1 -> LM_Fus_BLRearPath1Info/1(LM_FusBLFntPath1Quality)
  LM_FusBLRearPath1C0/1 -> LM_Fus_BLRearPath1Info/2(LM_FusBLFntPath1C0), LM_Fus_BLFntPath2Info/1(LM_FusBLRearPath1C0)
  LM_FusBLRearPath1C1/1 -> LM_Fus_BLRearPath1Info/3(LM_FusBLFntPath1C1), LM_Fus_BLFntPath2Info/2(LM_FusBLRearPath1C1)
  LM_FusBLRearPath1C2/1 -> LM_Fus_BLRearPath1Info/4(LM_FusBLFntPath1C2), LM_Fus_BLFntPath2Info/3(LM_FusBLRearPath1C2)
  LM_FusBLRearPath1C3/1 -> LM_Fus_BLRearPath1Info/5(LM_FusBLFntPath1C3), LM_Fus_BLFntPath2Info/4(LM_FusBLRearPath1C3)
  LM_FusBLRearPath2C0BefAduj/1 -> LM_Fus_BLFntPath2Info/6(LM_FusBLFntPath2C0BefAduj)
  LM_FusBLRearPath2C1/1 -> LM_Fus_BLFntPath2Info/7(LM_FusBLRearPath2C1), LM_Fus_BLFntPath3Info/2(LM_FusBLFntPath2C1)
  LM_FusBLRearPath2C2/1 -> LM_Fus_BLFntPath2Info/8(LM_FusBLRearPath2C2), LM_Fus_BLFntPath3Info/3(LM_FusBLFntPath2C2)
  LM_FusBLRearPath2C3/1 -> LM_Fus_BLFntPath2Info/9(LM_FusBLRearPath2C3), LM_Fus_BLFntPath3Info/4(LM_FusBLFntPath2C3)
  LM_FusBLRearPath2Quality/1 -> LM_Fus_BLFntPath2Info/5(LM_FusBLRearPath2Quality)
  LM_RearPath1Dis/1 -> LM_Fus_BLFntPath2Info/10(LM_RearPath1Dis)
  LM_FusBLRearPath3C0BefAduj/1 -> LM_Fus_BLFntPath3Info/5(LM_FusBLFntPath3C0BefAduj)
  LM_FusBRearPath3C1/1 -> LM_Fus_BLFntPath3Info/6(LM_FusBLFntPath3C1)
  LM_FusBLRearPath3C2/1 -> LM_Fus_BLFntPath3Info/7(LM_FusBLFntPath3C2)
  LM_FusBLRearPath3C3/1 -> LM_Fus_BLFntPath3Info/8(LM_FusBLFntPath3C3)
  LM_FusBLRearPath3Quality/1 -> LM_Fus_BLFntPath3Info/9(LM_FusBLFntPath3Quality)
  LM_RearPath2Dis/1 -> LM_Fus_BLFntPath3Info/10(LM_FntPath2Dis)
  LM_Fus_BLRearPath1Info/1(LM_FusBLRearPath1C0Adju) -> LM_FusBLRearPath1C0Adju/1
  LM_Fus_BLRearPath1Info/2(LM_FusBLRearPath1C1Adju) -> LM_FusBLRearPath1C1Adju/1
  LM_Fus_BLRearPath1Info/3(LM_FusBLRearPath1C2Adju) -> LM_FusBLRearPath1C2Adju/1
  LM_Fus_BLRearPath1Info/4(LM_FusBLRearPath1C3Adju) -> LM_FusBLRearPath1C3Adju/1
  LM_Fus_BLRearPath1Info/5(LM_FusBLRearPath1QualityAdju) -> LM_FusBLRearPath1QualityAdju/1
  LM_Fus_BLFntPath2Info/1(LM_FusBLRearPath2C0Adju) -> LM_FusBLRearPath2C0Adju/1, [LM_FusBLRearPath2C0Adju]
  LM_Fus_BLFntPath2Info/2(LM_FusBLRearPath2C1Adju) -> LM_FusBLRearPath2C1Adju/1
  LM_Fus_BLFntPath2Info/3(LM_FusBLRearPath2C2Adju) -> LM_FusBLRearPath2C2Adju/1
  LM_Fus_BLFntPath2Info/4(LM_FusBLRearPath2C3Adju) -> LM_FusBLRearPath2C3Adju/1
  LM_Fus_BLFntPath2Info/5(LM_FusBLRearPath2QualityAdju) -> LM_FusBLRearPath2QualityAdju/1
  LM_Fus_BLFntPath3Info/1(LM_FusBLRearPath3C0Adju) -> LM_FusBLRearPath3C0Adju/1
  LM_Fus_BLFntPath3Info/2(LM_FusBLRearPath3C1Adju) -> LM_FusBLRearPath3C1Adju/1
  LM_Fus_BLFntPath3Info/3(LM_FusBLRearPath3C2Adju) -> LM_FusBLRearPath3C2Adju/1
  LM_Fus_BLFntPath3Info/4(LM_FusBLRearPath3C3Adju) -> LM_FusBLRearPath3C3Adju/1
  LM_Fus_BLFntPath3Info/5(LM_FusBLRearPath3QualityAdju) -> LM_FusBLRearPath3QualityAdju/1
  [LM_FusBLRearPath2C0Adju] -> LM_Fus_BLFntPath3Info/1(LM_FusBLFntPath2C0Aduj)

== system PubIfDecisionLM_MDL/Subsystem2/LM_OTL/LM_OTL_MovObjTrajFit/LM_OTL_BufTPAssess/LM_OTL_BufTPInfoEva ==
  LM_ComBus : Inport
  LM_OTLBufTPVectBus : Inport  Port=2
  LM_OTLBufTPInfoBus : Inport  Port=3
  Bus Creator : BusCreator  Inputs=12
  Bus Selector1 : BusSelector  OutputSignals=LM_PathDisBus.LM_FntPath1Dis,LM_PathDisBus.LM_FntPath2Dis,LM_PathDisBus.LM_FntPath3Dis
  Bus Selector2 : BusSelector  OutputSignals=LM_OTLBufL1DxVect,LM_OTLBufL2DxVect,LM_OTLBufE1DxVect,LM_OTLBufE2DxVect,LM_OTLBufR1DxVect,LM_OTLBufR2DxVect
  Bus Selector3 : BusSelector  OutputSignals=LM_OTLBufSPPosInfo,LM_OTLBufEPPosInfo,LM_OTLBufLastSPPosInfo,LM_OTLBufLastEPPosInfo
  Constant : Constant  Value=P_LM_OTLBufTPInfoEvaFactor  OutDataTypeStr=single
  MATLAB Function : MATLAB Function  TreatAsAtomicUnit=on
  LM_OTLBufValid : Outport
  wires:
  Constant/1 -> MATLAB Function/14(P_LM_OTLBufTPInfoEvaFactor)
  LM_ComBus/1 -> Bus Selector1/1
  LM_OTLBufTPVectBus/1 -> Bus Selector2/1
  LM_OTLBufTPInfoBus/1 -> Bus Selector3/1
  Bus Selector2/1 -> MATLAB Function/1(LM_OTLBufL1DxVect)  "<LM_OTLBufL1DxVect>"
  Bus Selector2/2 -> MATLAB Function/2(LM_OTLBufL2DxVect)  "<LM_OTLBufL2DxVect>"
  Bus Selector2/3 -> MATLAB Function/3(LM_OTLBufE1DxVect)  "<LM_OTLBufE1DxVect>"
  Bus Selector2/4 -> MATLAB Function/4(LM_OTLBufE2DxVect)  "<LM_OTLBufE2DxVect>"
  Bus Selector2/5 -> MATLAB Function/5(LM_OTLBufR1DxVect)  "<LM_OTLBufR1DxVect>"
  Bus Selector2/6 -> MATLAB Function/6(LM_OTLBufR2DxVect)  "<LM_OTLBufR2DxVect>"
  Bus Selector3/1 -> MATLAB Function/7(LM_OTLBufSPPosInfo)  "<LM_OTLBufSPPosInfo>"
  Bus Selector3/2 -> MATLAB Function/8(LM_OTLBufEPPosInfo)  "<LM_OTLBufEPPosInfo>"
  Bus Selector3/3 -> MATLAB Function/9(LM_OTLBufLastSPPosInfo)  "<LM_OTLBufLastSPPosInfo>"
  Bus Selector3/4 -> MATLAB Function/10(LM_OTLBufLastEPPosInfo)  "<LM_OTLBufLastEPPosInfo>"
  Bus Selector1/1 -> MATLAB Function/11(LM_FntPath1Dis)  "<LM_FntPath1Dis>"
  Bus Selector1/2 -> MATLAB Function/12(LM_FntPath2Dis)  "<LM_FntPath2Dis>"
  Bus Selector1/3 -> MATLAB Function/13(LM_FntPath3Dis)  "<LM_FntPath3Dis>"
  Bus Creator/1 -> LM_OTLBufValid/1  "LM_OTLBufValid"
  MATLAB Function/1(LM_OTLBufL1LastValidInfo) -> Bus Creator/1  "LM_OTLBufL1LastValid"
  MATLAB Function/2(LM_OTLBufL2LastValidInfo) -> Bus Creator/2  "LM_OTLBufL2LastValid"
  MATLAB Function/3(LM_OTLBufE1LastValidInfo) -> Bus Creator/3  "LM_OTLBufE1LastValid"
  MATLAB Function/4(LM_OTLBufE2LastValidInfo) -> Bus Creator/4  "LM_OTLBufE2LastValid"
  MATLAB Function/5(LM_OTLBufR1LastValidInfo) -> Bus Creator/5  "LM_OTLBufR1LastValid"
  MATLAB Function/6(LM_OTLBufR2LastValidInfo) -> Bus Creator/6  "LM_OTLBufR2LastValid"
  MATLAB Function/7(LM_OTLBufL1ValidInfo) -> Bus Creator/7  "LM_OTLBufL1Valid"
  MATLAB Function/8(LM_OTLBufL2ValidInfo) -> Bus Creator/8  "LM_OTLBufL2Valid"
  MATLAB Function/9(LM_OTLBufE1ValidInfo) -> Bus Creator/9  "LM_OTLBufE1Valid"
  MATLAB Function/10(LM_OTLBufE2ValidInfo) -> Bus Creator/10  "LM_OTLBufE2Valid"
  MATLAB Function/11(LM_OTLBufR1ValidInfo) -> Bus Creator/11  "LM_OTLBufR1Valid"
  MATLAB Function/12(LM_OTLBufR2ValidInfo) -> Bus Creator/12  "LM_OTLBufR2Valid"

== system PubIfDecisionLM_MDL/Subsystem2/LM_OTL/LM_OTL_MovObjTrajFit/LM_OTL_BufTPAssess/LM_OTL_BufTrajEva ==
  LM_OTLBufValid : Inport
  LM_PathDisBus : Inport  Port=2
  LM_OTLBufTPVectBus : Inport  Port=3
  ILM_OTLBufTPInfoBus : Inport  Port=4
  Bus Creator : BusCreator  Inputs=48
  Subsystem : Subsystem
  Subsystem1 : Subsystem
  Subsystem10 : Subsystem
  Subsystem11 : Subsystem
  Subsystem2 : Subsystem
  Subsystem3 : Subsystem
  Subsystem4 : Subsystem
  Subsystem5 : Subsystem
  Subsystem6 : Subsystem
  Subsystem7 : Subsystem
  Subsystem8 : Subsystem
  Subsystem9 : Subsystem
  LM_OTL_BufTrajFlg : Outport
  wires:
  LM_OTLBufValid/1 -> Subsystem3/1(LM_OTLBufValid), Subsystem4/1(LM_OTLBufValid), Subsystem5/1(LM_OTLBufValid), Subsystem/1(LM_OTLBufValid), Subsystem11/1(LM_OTLBufValid), Subsystem10/1(LM_OTLBufValid), Subsystem9/1(LM_OTLBufValid), Subsystem8/1(LM_OTLBufValid), Subsystem7/1(LM_OTLBufValid), Subsystem6/1(LM_OTLBufValid), Subsystem2/1(LM_OTLBufValid), Subsystem1/1(LM_OTLBufValid)
  LM_OTLBufTPVectBus/1 -> Subsystem3/2(LM_OTLBufTPVectBus), Subsystem4/2(LM_OTLBufTPVectBus), Subsystem5/2(LM_OTLBufTPVectBus), Subsystem11/2(LM_OTLBufTPVectBus), Subsystem10/2(LM_OTLBufTPVectBus), Subsystem9/2(LM_OTLBufTPVectBus), Subsystem8/2(LM_OTLBufTPVectBus), Subsystem7/2(LM_OTLBufTPVectBus), Subsystem6/2(LM_OTLBufTPVectBus), Subsystem/2(LM_OTLBufTPVectBus), Subsystem2/2(LM_OTLBufTPVectBus), Subsystem1/2(LM_OTLBufTPVectBus)
  LM_PathDisBus/1 -> Subsystem3/4(LM_PathDisBus), Subsystem4/4(LM_PathDisBus), Subsystem5/4(LM_PathDisBus), Subsystem11/4(LM_PathDisBus), Subsystem10/4(LM_PathDisBus), Subsystem9/4(LM_PathDisBus), Subsystem8/4(LM_PathDisBus), Subsystem7/4(LM_PathDisBus), Subsystem6/4(LM_PathDisBus), Subsystem/4(LM_PathDisBus), Subsystem2/4(LM_PathDisBus), Subsystem1/4(LM_PathDisBus)
  Subsystem1/2(LM_OTLBufL1LastFlg) -> Bus Creator/2  "LM_OTLBufL1LastFlg"
  Subsystem1/1(LM_OTLBufL1LastOffset) -> Bus Creator/1  "LM_OTLBufL1LastOffset"
  Subsystem2/1(LM_OTLBufL1Offset) -> Bus Creator/5  "LM_OTLBufL1Offset"
  Subsystem2/2(LM_OTLBufL1Flg) -> Bus Creator/6  "LM_OTLBufL1Flg"
  Subsystem3/1(LM_OTLBufL2LastOffset) -> Bus Creator/9  "LM_OTLBufL2LastOffset"
  Subsystem3/2(LM_OTLBufL2LastFlg) -> Bus Creator/10  "LM_OTLBufL2LastFlg"
  Subsystem4/1(LM_OTLBufL2Offset) -> Bus Creator/13  "LM_OTLBufL2Offset"
  Subsystem4/2(LM_OTLBufL2Flg) -> Bus Creator/14  "LM_OTLBufL2Flg"
  Subsystem5/1(LM_OTLBufE1LastOffset) -> Bus Creator/17  "LM_OTLBufE1LastOffset"
  Subsystem5/2(LM_OTLBufE1LastFlg) -> Bus Creator/18  "LM_OTLBufE1LastFlg"
  Subsystem/1(LM_OTLBufE1Offset) -> Bus Creator/21  "LM_OTLBufE1Offset"
  Subsystem/2(LM_OTLBufE1Flg) -> Bus Creator/22  "LM_OTLBufE1Flg"
  Subsystem6/2(LM_OTLBufE2LastFlg) -> Bus Creator/26  "LM_OTLBufE2LastFlg"
  Subsystem6/1(LM_OTLBufE2LastOffset) -> Bus Creator/25  "LM_OTLBufE2LastOffset"
  ILM_OTLBufTPInfoBus/1 -> Subsystem3/3(ILM_OTLBufTPInfoBus), Subsystem4/3(ILM_OTLBufTPInfoBus), Subsystem5/3(ILM_OTLBufTPInfoBus), Subsystem11/3(ILM_OTLBufTPInfoBus), Subsystem10/3(ILM_OTLBufTPInfoBus), Subsystem9/3(ILM_OTLBufTPInfoBus), Subsystem8/3(ILM_OTLBufTPInfoBus), Subsystem7/3(ILM_OTLBufTPInfoBus), Subsystem6/3(ILM_OTLBufTPInfoBus), Subsystem/3(ILM_OTLBufTPInfoBus), Subsystem2/3(ILM_OTLBufTPInfoBus), Subsystem1/3(ILM_OTLBufTPInfoBus)
  Subsystem7/1(LM_OTLBufE2Offset) -> Bus Creator/29  "LM_OTLBufE2Offset"
  Subsystem7/2(LM_OTLBufE2Flg) -> Bus Creator/30  "LM_OTLBufE2Flg"
  Subsystem8/1(LM_OTLBufR1LastOffset) -> Bus Creator/33  "LM_OTLBufR1LastOffset"
  Subsystem8/2(LM_OTLBufR1LastFlg) -> Bus Creator/34  "LM_OTLBufR1LastFlg"
  Subsystem9/1(LM_OTLBufR1Offset) -> Bus Creator/37  "LM_OTLBufR1Offset"
  Subsystem9/2(LM_OTLBufR1Flg) -> Bus Creator/38  "LM_OTLBufR1Flg"
  Subsystem10/1(LM_OTLBufR2LastOffset) -> Bus Creator/41  "LM_OTLBufR2LastOffset"
  Subsystem10/2(LM_OTLBufR2LastFlg) -> Bus Creator/42  "LM_OTLBufR2LastFlg"
  Subsystem11/1(LM_OTLBufR2Offset) -> Bus Creator/45  "LM_OTLBufR2Offset"
  Subsystem11/2(LM_OTLBufR2Flg) -> Bus Creator/46  "LM_OTLBufR2Flg"
  Bus Creator/1 -> LM_OTL_BufTrajFlg/1
  Subsystem1/3(LM_OTLBufL1TpLastValidNum) -> Bus Creator/3  "LM_OTLBufL1TpLastValidNum"
  Subsystem1/4(LM_OTLBufL1SPLastValidPos) -> Bus Creator/4  "LM_OTLBufL1SPLastValidPos"
  Subsystem2/3(LM_OTLBufL1TpValidNum) -> Bus Creator/7  "LM_OTLBufL1TpValidNum"
  Subsystem2/4(LM_OTLBufL1SPValidPos) -> Bus Creator/8  "LM_OTLBufL1SPValidPos"
  Subsystem3/3(LM_OTLBufL2TpLastValidNum) -> Bus Creator/11  "LM_OTLBufL2TpLastValidNum"
  Subsystem3/4(LM_OTLBufL2SPLastValidPos) -> Bus Creator/12  "LM_OTLBufL2SPLastValidPos"
  Subsystem4/3(LM_OTLBufL2TpValidNum) -> Bus Creator/15  "LM_OTLBufL2TpValidNum"
  Subsystem4/4(LM_OTLBufL2SPValidPos) -> Bus Creator/16  "LM_OTLBufL2SPValidPos"
  Subsystem5/3(LM_OTLBufE1TpLastValidNum) -> Bus Creator/19  "LM_OTLBufE1TpLastValidNum"
  Subsystem5/4(LM_OTLBufE1SPLastValidPos) -> Bus Creator/20  "LM_OTLBufE1SPLastValidPos"
  Subsystem/3(LM_OTLBufE1TpValidNum) -> Bus Creator/23  "LM_OTLBufE1TpValidNum"
  Subsystem/4(LM_OTLBufE1SPValidPos) -> Bus Creator/24  "LM_OTLBufE1SPValidPos"
  Subsystem6/3(LM_OTLBufE2TpLastValidNum) -> Bus Creator/27  "LM_OTLBufE2TpLastValidNum"
  Subsystem6/4(LM_OTLBufE2SPLastValidPos) -> Bus Creator/28  "LM_OTLBufE2SPLastValidPos"
  Subsystem7/3(LM_OTLBufE2TpValidNum) -> Bus Creator/31  "LM_OTLBufE2TpValidNum"
  Subsystem7/4(LM_OTLBufE2SPValidPos) -> Bus Creator/32  "LM_OTLBufE2SPValidPos"
  Subsystem8/3(LM_OTLBufR1TpLastValidNum) -> Bus Creator/35  "LM_OTLBufR1TpLastValidNum"
  Subsystem8/4(LM_OTLBufR1SPLastValidPos) -> Bus Creator/36  "LM_OTLBufR1SPLastValidPos"
  Subsystem9/3(LM_OTLBufR1TpValidNum) -> Bus Creator/39  "LM_OTLBufR1TpValidNum"
  Subsystem9/4(LM_OTLBufR1SPValidPos) -> Bus Creator/40  "LM_OTLBufR1SPValidPos"
  Subsystem10/3(LM_OTLBufR2TpLastValidNum) -> Bus Creator/43  "LM_OTLBufR2TpLastValidNum"
  Subsystem10/4(LM_OTLBufR2SPLastValidPos) -> Bus Creator/44  "LM_OTLBufR2SPLastValidPos"
  Subsystem11/3(LM_OTLBufR2TpValidNum) -> Bus Creator/47  "LM_OTLBufR2TpValidNum"
  Subsystem11/4(LM_OTLBufR2SPValidPos) -> Bus Creator/48  "LM_OTLBufR2SPValidPos"

== system PubIfDecisionLM_MDL/Subsystem2/LM_OTL/LM_OTL_MovObjTrajRecord3/LM_OTL_BufRcdObjLostJudge/LM_OTL_EgoLaRcdObjLostJudge ==
  Object_ID : Inport  BusOutputAsStruct=on
  LM_OTLRcdObjIDVectK1 : Inport  Port=2
  LM_OTLInterestObjIndexVect : Inport  Port=3
  Bus Selector : BusSelector  OutputSignals=LM_OTLCurEgoLaObj1Index,LM_OTLCurEgoLaObj2Index
  Bus Selector1 : BusSelector  OutputSignals=LM_OTLBufObjIDInfo.LM_OTLBufE1ObjID,LM_OTLBufObjIDInfo.LM_OTLBufE2ObjID
  Compare To Zero : simulink/Logic and Bit Operations/Compare To Zero  relop===  OutDataTypeStr=boolean
  Compare To Zero1 : simulink/Logic and Bit Operations/Compare To Zero  relop===  OutDataTypeStr=boolean
  Compare To Zero2 : simulink/Logic and Bit Operations/Compare To Zero  relop=~=  OutDataTypeStr=boolean
  Compare To Zero3 : simulink/Logic and Bit Operations/Compare To Zero  relop===  OutDataTypeStr=boolean
  Constant : Constant  OutDataTypeStr=uint8
  Constant1 : Constant  OutDataTypeStr=uint8
  Constant2 : Constant  Value=0  OutDataTypeStr=boolean
  Constant3 : Constant  Value=0  OutDataTypeStr=boolean
  Constant4 : Constant  Value=0  OutDataTypeStr=uint8
  Index Vector2 : MultiPortSwitch  Inputs=1
  Index Vector3 : MultiPortSwitch  Inputs=1
  Logical Operator : Logic  Operator=OR  AllPortsSameDT=off  OutDataTypeStr=boolean
  Logical Operator1 : Logic  Operator=OR  AllPortsSameDT=off  OutDataTypeStr=boolean
  Logical Operator2 : Logic  Operator=NOT  AllPortsSameDT=off  OutDataTypeStr=boolean
  Logical Operator3 : Logic  Operator=NOT  AllPortsSameDT=off  OutDataTypeStr=boolean
  Relational Operator{,1..3} (4 alike) : RelationalOperator  Operator===  OutDataTypeStr=boolean  RndMeth=Simplest
  Switch{,1..5} (6 alike) : Switch  Criteria=u2 ~= 0
  LM_OTLBufEgo1ObjLostFlg : Outport
  LM_OTLBufEgo2ObjLostFlg : Outport  Port=2
  wires:
  Logical Operator/1 -> Logical Operator3/1
  Logical Operator1/1 -> Logical Operator2/1
  Relational Operator3/1 -> Logical Operator1/2
  Relational Operator1/1 -> Logical Operator1/1
  Relational Operator2/1 -> Logical Operator/2
  Logical Operator2/1 -> Switch4/1
  Relational Operator/1 -> Logical Operator/1
  Switch2/1 -> Index Vector3/1
  Bus Selector1/2 -> Relational Operator1/2, Relational Operator3/2, Compare To Zero2/1  "<LM_OTLBufE2ObjID>"
  Bus Selector/1 -> Switch/3, Compare To Zero/1  "<LM_OTLCurEgoLaObj1Index>"
  Switch3/1 -> Relational Operator3/1, Relational Operator2/1  "LM_Ego2ObjID"
  Bus Selector1/1 -> Compare To Zero3/1, Relational Operator/2, Relational Operator2/2  "<LM_OTLBufE1ObjID>"
  Constant/1 -> Switch/1
  Object_ID/1 -> Index Vector3/2, Index Vector2/2
  Logical Operator3/1 -> Switch5/3
  Switch1/1 -> Relational Operator1/1, Relational Operator/1  "LM_Ego1ObjID"
  Switch/1 -> Index Vector2/1
  Compare To Zero/1 -> Switch/2, Switch1/2
  LM_OTLInterestObjIndexVect/1 -> Bus Selector/1
  Constant4/1 -> Switch3/1, Switch1/1
  Index Vector2/1 -> Switch1/3
  Bus Selector/2 -> Switch2/3, Compare To Zero1/1  "<LM_OTLCurEgoLaObj2Index>"
  Compare To Zero1/1 -> Switch3/2, Switch2/2
  Index Vector3/1 -> Switch3/3  "LM_Le2ObjID"
  Constant1/1 -> Switch2/1
  LM_OTLRcdObjIDVectK1/1 -> Bus Selector1/1
  Switch4/1 -> LM_OTLBufEgo2ObjLostFlg/1  "LM_OTLBufEgo2ObjLostFlg"
  Compare To Zero2/1 -> Switch4/2
  Constant2/1 -> Switch4/3
  Compare To Zero3/1 -> Switch5/2
  Switch5/1 -> LM_OTLBufEgo1ObjLostFlg/1  "LM_OTLBufEgo1ObjLostFlg"
  Constant3/1 -> Switch5/1

== system PubIfDecisionLM_MDL/Subsystem2/LM_OTL/LM_OTL_MovObjTrajRecord3/LM_OTL_BufRcdObjLostJudge/LM_OTL_LeLaRcdObjLostJudge ==
  Object_ID : Inport  BusOutputAsStruct=on
  LM_OTLRcdObjIDVectK1 : Inport  Port=2
  LM_OTLInterestObjIndexVect : Inport  Port=3
  Bus Selector : BusSelector  OutputSignals=LM_OTLCurLeLaObj1Index,LM_OTLCurLeLaObj2Index
  Bus Selector1 : BusSelector  OutputSignals=LM_OTLBufObjIDInfo.LM_OTLBufL1ObjID,LM_OTLBufObjIDInfo.LM_OTLBufL2ObjID
  Compare To Zero : simulink/Logic and Bit Operations/Compare To Zero  relop===  OutDataTypeStr=boolean
  Compare To Zero1 : simulink/Logic and Bit Operations/Compare To Zero  relop===  OutDataTypeStr=boolean
  Compare To Zero2 : simulink/Logic and Bit Operations/Compare To Zero  relop=~=  OutDataTypeStr=boolean
  Compare To Zero3 : simulink/Logic and Bit Operations/Compare To Zero  relop===  OutDataTypeStr=boolean
  Constant : Constant  OutDataTypeStr=uint8
  Constant1 : Constant  OutDataTypeStr=uint8
  Constant2 : Constant  Value=0  OutDataTypeStr=boolean
  Constant3 : Constant  Value=0  OutDataTypeStr=boolean
  Constant4 : Constant  Value=0  OutDataTypeStr=uint8
  Index Vector2 : MultiPortSwitch  Inputs=1
  Index Vector3 : MultiPortSwitch  Inputs=1
  Logical Operator : Logic  Operator=OR  AllPortsSameDT=off  OutDataTypeStr=boolean
  Logical Operator1 : Logic  Operator=OR  AllPortsSameDT=off  OutDataTypeStr=boolean
  Logical Operator2 : Logic  Operator=NOT  AllPortsSameDT=off  OutDataTypeStr=boolean
  Logical Operator3 : Logic  Operator=NOT  AllPortsSameDT=off  OutDataTypeStr=boolean
  Relational Operator{,1..3} (4 alike) : RelationalOperator  Operator===  OutDataTypeStr=boolean  RndMeth=Simplest
  Switch{,1..5} (6 alike) : Switch  Criteria=u2 ~= 0
  LM_OTLBufLe1ObjLostFlg : Outport
  LM_OTLBufLe2ObjLostFlg : Outport  Port=2
  wires:
  Constant3/1 -> Switch5/1
  Switch5/1 -> LM_OTLBufLe1ObjLostFlg/1  "LM_OTLBufLe1ObjLostFlg"
  Compare To Zero3/1 -> Switch5/2
  Constant2/1 -> Switch4/3
  Compare To Zero2/1 -> Switch4/2
  Switch4/1 -> LM_OTLBufLe2ObjLostFlg/1  "LM_OTLBufLe2ObjLostFlg"
  LM_OTLRcdObjIDVectK1/1 -> Bus Selector1/1
  Constant1/1 -> Switch2/1
  Index Vector3/1 -> Switch3/3  "LM_Le2ObjID"
  Compare To Zero1/1 -> Switch2/2, Switch3/2
  Bus Selector/2 -> Compare To Zero1/1, Switch2/3  "<LM_OTLCurLeLaObj2Index>"
  Index Vector2/1 -> Switch1/3
  Constant4/1 -> Switch1/1, Switch3/1
  LM_OTLInterestObjIndexVect/1 -> Bus Selector/1
  Compare To Zero/1 -> Switch1/2, Switch/2
  Switch/1 -> Index Vector2/1
  Switch1/1 -> Relational Operator/1, Relational Operator1/1  "LM_Le1ObjID"
  Logical Operator3/1 -> Switch5/3
  Object_ID/1 -> Index Vector2/2, Index Vector3/2
  Constant/1 -> Switch/1
  Bus Selector1/1 -> Relational Operator2/2, Relational Operator/2, Compare To Zero3/1  "<LM_OTLBufL1ObjID>"
  Switch3/1 -> Relational Operator2/1, Relational Operator3/1  "LM_Le2ObjID"
  Bus Selector/1 -> Compare To Zero/1, Switch/3  "<LM_OTLCurLeLaObj1Index>"
  Bus Selector1/2 -> Compare To Zero2/1, Relational Operator3/2, Relational Operator1/2  "<LM_OTLBufL2ObjID>"
  Switch2/1 -> Index Vector3/1
  Relational Operator/1 -> Logical Operator/1
  Logical Operator2/1 -> Switch4/1
  Relational Operator2/1 -> Logical Operator/2
  Relational Operator1/1 -> Logical Operator1/1
  Relational Operator3/1 -> Logical Operator1/2
  Logical Operator1/1 -> Logical Operator2/1
  Logical Operator/1 -> Logical Operator3/1
